simulink model "multiportswitch_vect_test"  (Simulink 8.4)
settings: Solver=VariableStepDiscrete  StartTime=0.0  StopTime=0  MaxStep=1  RelTol=1e-3
settings Model: Creator=arnaud  LastModifiedBy=arnaud
settings DataIOCC: SaveFormat=Structure  SignalLoggingSaveFormat=Dataset
settings OptimizationCC: ExpressionDepthLimit=128
settings DebuggingCC: UnderspecifiedInitializationDetection=Simplified  MergeDetectMultiDrivingBlocksExec=error  FcnCallInpInsideContextMsg=EnableAllAsError  StateNameClashWarn=none
settings GRTTargetCC: CombineOutputUpdateFcns=on  GRTInterface=off

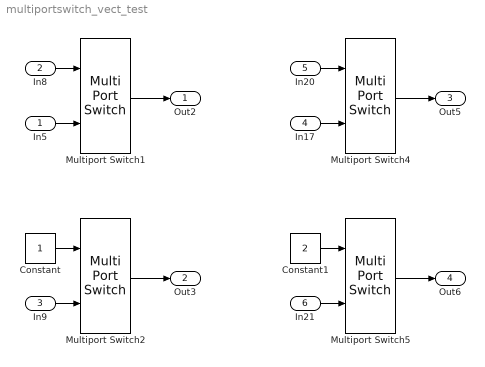
== system multiportswitch_vect_test ==
  In5 : Inport  PortDimensions=5
  In8 : Inport  Port=2  OutDataTypeStr=int8  PortDimensions=1
  In9 : Inport  Port=3  PortDimensions=1
  In17 : Inport  Port=4  PortDimensions=9
  In20 : Inport  Port=5  OutDataTypeStr=int8  PortDimensions=1
  In21 : Inport  Port=6  PortDimensions=4
  Constant : Constant  OutDataTypeStr=uint8
  Constant1 : Constant  Value=2  OutDataTypeStr=uint32
  Multiport Switch1 : MultiPortSwitch  DataPortOrder=Zero-based contiguous  Inputs=1  DataPortIndices={1,[2,3]}  DataPortForDefault=Additional data port  DiagnosticForDefault=Warning
  Multiport Switch2 : MultiPortSwitch  Inputs=1  DataPortIndices={1,[2,3]}  DataPortForDefault=Additional data port  DiagnosticForDefault=Warning
  Multiport Switch4 : MultiPortSwitch  DataPortOrder=Zero-based contiguous  Inputs=1  DataPortIndices={1,[2,3]}  DiagnosticForDefault=Warning
  Multiport Switch5 : MultiPortSwitch  Inputs=1  DataPortIndices={1,[2,3]}  DiagnosticForDefault=Warning
  Out2 : Outport
  Out3 : Outport  Port=2
  Out5 : Outport  Port=3
  Out6 : Outport  Port=4
  wires:
  Multiport Switch1/1 -> Out2/1
  In5/1 -> Multiport Switch1/2
  In8/1 -> Multiport Switch1/1
  Multiport Switch2/1 -> Out3/1
  In9/1 -> Multiport Switch2/2
  Constant/1 -> Multiport Switch2/1
  Multiport Switch4/1 -> Out5/1
  In17/1 -> Multiport Switch4/2
  In20/1 -> Multiport Switch4/1
  Multiport Switch5/1 -> Out6/1
  In21/1 -> Multiport Switch5/2
  Constant1/1 -> Multiport Switch5/1
